simulink library "drag_library_masked"  (Simulink 7.5)
settings: Solver=ode45  SolverMode=SingleTasking  StartTime=0.0  StopTime=10.0  RelTol=1e-3
libraries: simulink x1, aerolibatmos2 x1
settings Model: Creator=wcampbel  LastModifiedBy=wcampbel

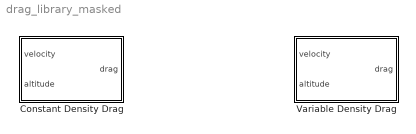
== system drag_library_masked ==
  Constant Density Drag : Subsystem  mask(Constant Density Drag Model){rho=1.2, Cd=0.333, A=1.5}
      mask prompts: rho "Air Density [kg/m^3]"; Cd "Drag Coefficient [N/A]"; A "Reference Area [m^2]"
      mask help: Applies the equation D = -0.5*rho*Cd*A*V^2. V is designed to be a velocity vector of length 3.
  Variable Density Drag : Subsystem  mask(Variable Density Drag Model){Cd=0.333, A=1.5}
      mask prompts: Cd "Drag Coefficient [N/A]"; A "Reference Area [m^2]"
      mask help: Applies the equation D = -0.5*rho*Cd*A*V^2. V is designed to be a velocity vector of length 3.

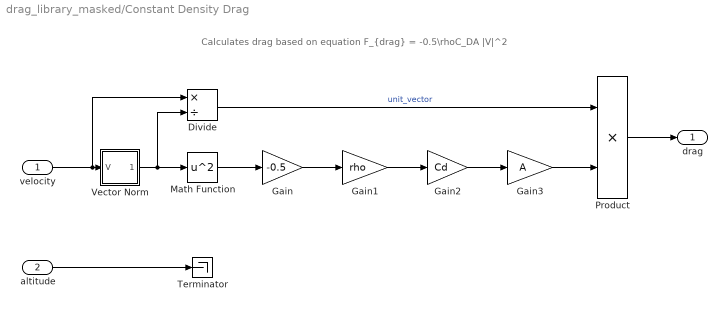
== system drag_library_masked/Constant Density Drag ==
  note: Calculates drag based on equation F_{drag} = -0.5\rhoC_DA |V|^2
  velocity : Inport  OutDataType=sfix(16)  OutScaling=2^0
  altitude : Inport  Port=2  OutDataType=sfix(16)  OutScaling=2^0
  Divide : Product  Inputs=*/  OutDataType=sfix(16)  OutScaling=2^-10
  Gain : Gain  Gain=-0.5  ParameterDataType=sfix(16)  ParameterScaling=2^0  OutDataType=sfix(16)  OutScaling=2^0
  Gain1 : Gain  Gain=rho  ParameterDataType=sfix(16)  ParameterScaling=2^0  OutDataType=sfix(16)  OutScaling=2^0
  Gain2 : Gain  Gain=Cd  ParameterDataType=sfix(16)  ParameterScaling=2^0  OutDataType=sfix(16)  OutScaling=2^0
  Gain3 : Gain  Gain=A  ParameterDataType=sfix(16)  ParameterScaling=2^0  OutDataType=sfix(16)  OutScaling=2^0
  Math Function : Math  Operator=square  OutDataType=sfix(16)  OutScaling=2^0  SaturateOnIntegerOverflow=on
  Product : Product  OutDataType=sfix(16)  OutScaling=2^0  RndMeth=Zero
  Terminator : Terminator
  Vector Norm : Subsystem
      mask Type: Vector Norm
      mask Description: Calculates the magnitude of a vector of arbitrary length.
      mask Help:
      | Will Campbell
      | Senior Application Engineer
      | The MathWorks, Inc.
      | 14 Nov 2007
      mask Display: disp('|\bfV|','texmode','on')
  drag : Outport  OutDataType=sfix(16)  OutScaling=2^0
  wires:
  altitude/1 -> Terminator/1
  velocity/1 -> Vector Norm/1(V), Divide/1
  Vector Norm/1(norm) -> Math Function/1, Divide/2
  Gain/1 -> Gain1/1
  Gain1/1 -> Gain2/1
  Gain2/1 -> Gain3/1
  Math Function/1 -> Gain/1
  Divide/1 -> Product/1  "unit_vector"
  Gain3/1 -> Product/2
  Product/1 -> drag/1

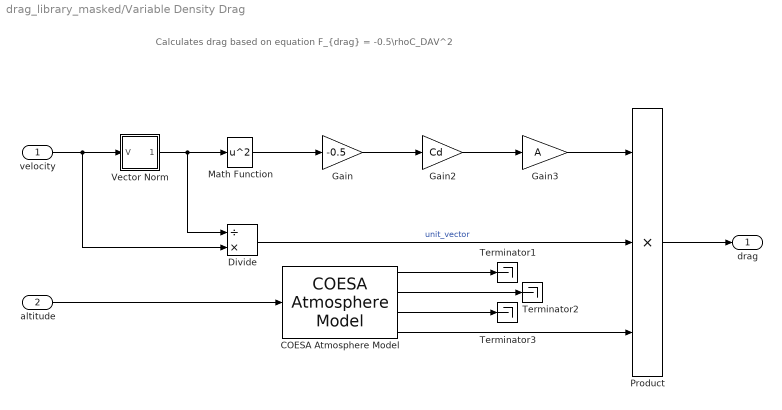
== system drag_library_masked/Variable Density Drag ==
  note: Calculates drag based on equation F_{drag} = -0.5\rhoC_DAV^2
  velocity : Inport  OutDataType=sfix(16)  OutScaling=2^0
  altitude : Inport  Port=2  OutDataType=sfix(16)  OutScaling=2^0
  COESA Atmosphere Model : aerolibatmos2/COESA Atmosphere Model  SystemSampleTime=-1  units=Metric (MKS)  spec=1976 COESA-extended U.S. Standard Atmosphere  model=Profile  profile_var=High temperature  profile_percent=1%  profile_alt=5 km (16404 ft)  envelope_var=High temperature  envelope_percent=1%  action=None
  Divide : Product  Inputs=/*  OutDataType=sfix(16)  OutScaling=2^-10
  Gain : Gain  Gain=-0.5  ParameterDataType=sfix(16)  ParameterScaling=2^0  OutDataType=sfix(16)  OutScaling=2^0
  Gain2 : Gain  Gain=Cd  ParameterDataType=sfix(16)  ParameterScaling=2^0  OutDataType=sfix(16)  OutScaling=2^0
  Gain3 : Gain  Gain=A  ParameterDataType=sfix(16)  ParameterScaling=2^0  OutDataType=sfix(16)  OutScaling=2^0
  Math Function : Math  Operator=square  OutDataType=sfix(16)  OutScaling=2^0  SaturateOnIntegerOverflow=on
  Product : Product  Inputs=3  OutDataType=sfix(16)  OutScaling=2^0  RndMeth=Zero
  Terminator1 : Terminator
  Terminator2 : Terminator
  Terminator3 : Terminator
  Vector Norm : Subsystem
      mask Type: Vector Norm
      mask Description: Calculates the magnitude of a vector of arbitrary length.
      mask Help:
      | Will Campbell
      | Senior Application Engineer
      | The MathWorks, Inc.
      | 14 Nov 2007
      mask Display: disp('|\bfV|','texmode','on')
  drag : Outport  OutDataType=sfix(16)  OutScaling=2^0
  wires:
  altitude/1 -> COESA Atmosphere Model/1
  velocity/1 -> Divide/2, Vector Norm/1(V)
  Math Function/1 -> Gain/1
  Gain2/1 -> Gain3/1
  COESA Atmosphere Model/1 -> Terminator1/1
  COESA Atmosphere Model/2 -> Terminator2/1
  COESA Atmosphere Model/3 -> Terminator3/1
  Gain/1 -> Gain2/1
  Vector Norm/1(norm) -> Math Function/1, Divide/1
  Product/1 -> drag/1
  Gain3/1 -> Product/1
  Divide/1 -> Product/2  "unit_vector"
  COESA Atmosphere Model/4 -> Product/3

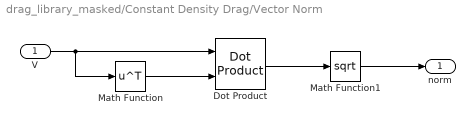
== system drag_library_masked/Constant Density Drag/Vector Norm ==
  V : Inport  OutDataType=sfix(16)  OutScaling=2^0
  Dot Product : simulink/Math Operations/Dot Product  InputSameDT=on  OutDataType=sfix(16)  OutScaling=2^-10  DoSatur=off
  Math Function : Math  Operator=transpose  OutDataType=sfix(16)  OutScaling=2^0  SaturateOnIntegerOverflow=on
  Math Function1 : Math  Operator=sqrt  OutDataType=sfix(16)  OutScaling=2^0  SaturateOnIntegerOverflow=on
  norm : Outport  OutDataType=sfix(16)  OutScaling=2^0
  wires:
  V/1 -> Dot Product/1, Math Function/1
  Math Function/1 -> Dot Product/2
  Dot Product/1 -> Math Function1/1
  Math Function1/1 -> norm/1

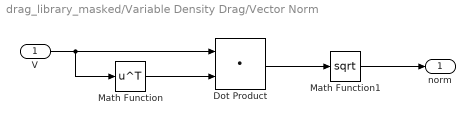
== system drag_library_masked/Variable Density Drag/Vector Norm ==
  V : Inport  OutDataType=sfix(16)  OutScaling=2^0
  Dot Product : DotProduct  OutDataType=sfix(16)  OutScaling=2^-10  InputSameDT=on  OutDataTypeStr=Inherit: Inherit via internal rule
  Math Function : Math  Operator=transpose  OutDataType=sfix(16)  OutScaling=2^0  SaturateOnIntegerOverflow=on
  Math Function1 : Math  Operator=sqrt  OutDataType=sfix(16)  OutScaling=2^0  SaturateOnIntegerOverflow=on
  norm : Outport  OutDataType=sfix(16)  OutScaling=2^0
  wires:
  Math Function1/1 -> norm/1
  Dot Product/1 -> Math Function1/1
  Math Function/1 -> Dot Product/2
  V/1 -> Math Function/1, Dot Product/1
